simulink model "SS_Part2"  (R2024b)
settings: Solver=FixedStepAuto  StartTime=0.0  StopTime=orbital_period  FixedStep=10  RelTol=1e-3
values from neighbouring files (symbols this model uses):
  Eul0_b_eci = Eul0_b_eci(:)    [Final_3.m]    (also in ORR_part4_script.m = [phi_b_eci_0; theta_b_eci_0; psi_b_eci_0]; Part2_TorqueFreeMotion.m = [phi_b_eci_0; theta_b_eci_0; psi_b_eci_0]; Part2_TorqueFreeMotion_SS.m = [phi_b_eci_0; theta_b_eci_0; psi_b_eci_0]; Part5_TorqueFreeMotion_SS.m = [phi_b_eci_0; theta_b_eci_0; psi_b_eci_0])
  q0_b_eci = q0_b_eci(:)    [Final_3.m]    (also in ORR_part4_script.m; Part2_TorqueFreeMotion.m = DCM_to_quat(C_b_ECI_0); Part2_TorqueFreeMotion_SS.m = DCM_to_quat(C_b_ECI_0); Part5_TorqueFreeMotion_SS.m = DCM_to_quat(C_b_ECI_0))
  T = T_c    [Final_3.m]    (also in ORR_part4_script.m; Part2_TorqueFreeMotion.m = [0;0;0]; Part2_TorqueFreeMotion_SS.m = [0;0;0]; Part5_TorqueFreeMotion_SS.m = [0;0;0])
  w0_b_eci = [0.001; -0.001; 0.002]    [Part2_TorqueFreeMotion.m]    (also in Part2_TorqueFreeMotion_SS.m; Part5_TorqueFreeMotion_SS.m)
undefined symbols (not defined in the file or in its folder): n
settings Model: Creator=emehiel  LastModifiedBy=dstan
settings SolverCC: AlgebraicLoopSolver=TrustRegion
settings DebuggingCC: UnconnectedInputMsg=warning  UnconnectedOutputMsg=warning  UnconnectedLineMsg=warning
settings ModelReferenceCC: EnableRefExpFcnMdlSchedulingChecks=on
settings RTWCC: GPUComputeCapability=3.5

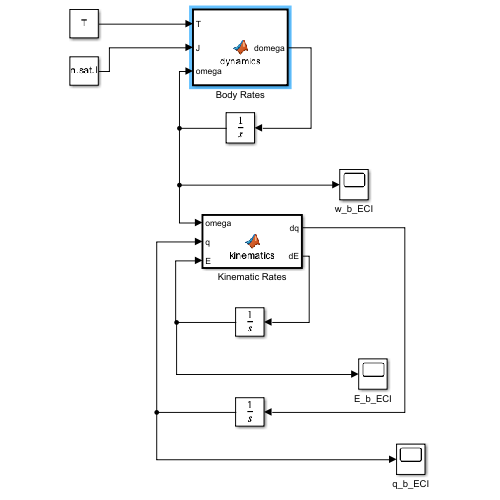
[thumbnail: Simulink's stored preview of the top-level diagram]
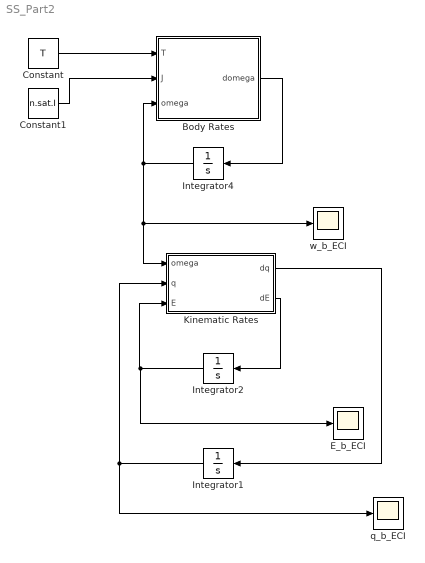
== system SS_Part2 ==
  Body Rates : MATLAB Function  TreatAsAtomicUnit=on
  Constant : Constant  Value=T
  Constant1 : Constant  Value=n.sat.I
  E_b_ECI : Scope
  Integrator1 : Integrator  InitialCondition=q0_b_eci
  Integrator2 : Integrator  InitialCondition=Eul0_b_eci
  Integrator4 : Integrator  InitialCondition=w0_b_eci
  Kinematic Rates : MATLAB Function  TreatAsAtomicUnit=on
  q_b_ECI : Scope
  w_b_ECI : Scope
  wires:
  Constant/1 -> Body Rates/1(T)
  Constant1/1 -> Body Rates/2(J)
  Body Rates/1(domega) -> Integrator4/1
  Integrator4/1 -> Body Rates/3(omega), w_b_ECI/1, Kinematic Rates/1(omega)
  Integrator2/1 -> E_b_ECI/1, Kinematic Rates/3(E)
  Integrator1/1 -> q_b_ECI/1, Kinematic Rates/2(q)
  Kinematic Rates/2(dE) -> Integrator2/1
  Kinematic Rates/1(dq) -> Integrator1/1

== matlab function SS_Part2/Kinematic Rates ==
  data: omega input; q input; dq output; E input; dE output
function [dq, dE] = kinematics(omega, q, E)
% column vecs
omega = omega(:);
q = q(:);
E = E(:);

% unpack euler angles
phi = E(1);
theta = E(2);
psi = E(3);

% unpack quat
eps = q(1:3);
eta = q(4);

% euler derivative
B = [1, sin(phi)*tan(theta),  cos(phi)*tan(theta);
     0, cos(phi),            -sin(phi);
     0, sin(phi)/cos(theta),  cos(phi)/cos(theta)];

dE = B * omega;

% quat derivative
dq = zeros(4,1);
dq(1:3) = 0.5 * ((eta*eye(3) + skew(eps)) * omega);
dq(4)   = -0.5 * (eps.' * omega);

end

== matlab function SS_Part2/Body Rates ==
  data: T input; J input; omega input; domega output
function domega = dynamics(T, J, omega)

%column vecs
omega = omega(:);
T = T(:);

domega = J \ (T - cross(omega, J*omega));
end
